simulink model "balancingController"  (Simulink 7.9)
settings: Solver=FixedStepDiscrete  StartTime=0.0  StopTime=60  FixedStep=Ts  RelTol=1e-3
InitFcn:
  | initBalancingController;
model workspace (MATLAB code in the model file):
  | Ts = 0.01;
undefined symbols (not defined in the file): DiscIntNeverNeededParam
libraries: WBCLibrary x12, simulink x2, dspsigops x2
settings Model: Creator=daniele  LastModifiedBy=morteza
settings DataIOCC: SignalLoggingSaveFormat=Dataset
settings SFSimCC: SimParseCustomCode=off
settings GRTTargetCC: CombineOutputUpdateFcns=off  GRTInterface=on

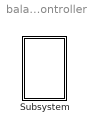
== system balancingController ==
  Subsystem : Subsystem  mask{robotName='icubGazeboSim', Ts=Ts, localName='dynamicBalancing'}
      mask prompts: robotName "robot name"; localName "module name"

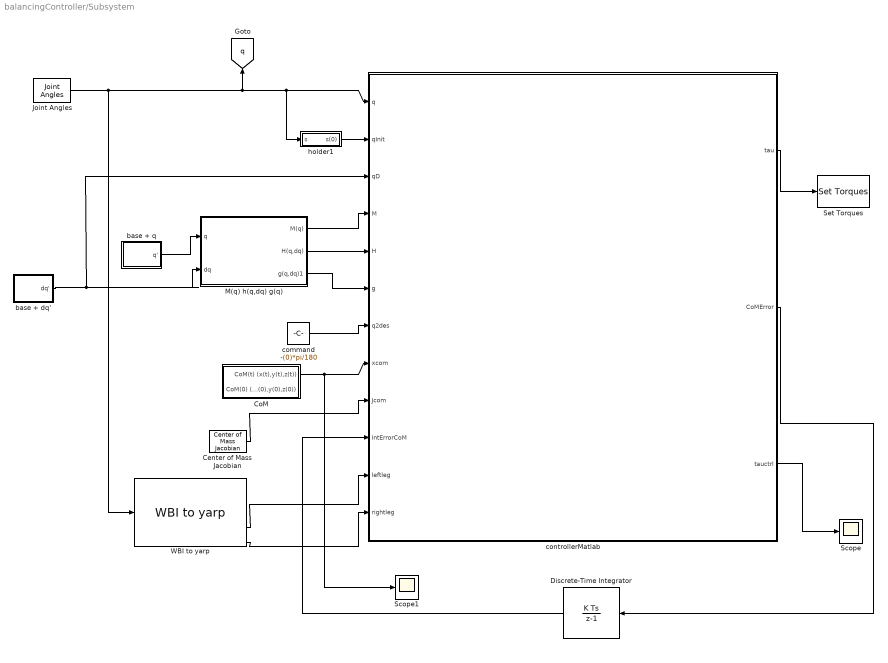
== system balancingController/Subsystem ==
  Center of Mass Jacobian : WBCLibrary/wholeBodyModel/Jacobians/Center of Mass Jacobian  robotName=robotName  localName=localName
  "CoM " : Subsystem
  Discrete-Time Integrator : DiscreteIntegrator  InitialCondition=[0 0 0]  SampleTime=Ts  ICPrevOutput=DiscIntNeverNeededParam  ICPrevScaledInput=DiscIntNeverNeededParam
  Joint Angles : WBCLibrary/wholeBodyStates/Joint Angles  robotName=robotName  localName=localName
  M(q) h(q,dq) g(q) : Subsystem
  Scope : Scope
      settings: YMin=16.125  YMax=16.325
  Scope1 : Scope
      settings: ShowLegends=on  YMin=-0.1  YMax=0.5
  Set Torques : WBCLibrary/wholeBodyActuators/Set Torques  val=6  robotName=robotName  localName=localName
  WBI to yarp : WBCLibrary/Utilities/WBI to yarp
  base + dq' : Subsystem
  base + q : Subsystem
  command : Constant  Value=-(0)*pi/180
  controllerMatlab : MATLAB Function  TreatAsAtomicUnit=on
  holder1 : Subsystem
  tag scope: q=global
  wires:
  Discrete-Time Integrator/1 -> controllerMatlab/10(IntErrorCoM)
  base + q/1(q') -> M(q) h(q,dq) g(q)/1(q)
  Joint Angles/1 -> [q], holder1/1(s), controllerMatlab/1(q), WBI to yarp/1
  controllerMatlab/2(CoMError) -> Discrete-Time Integrator/1
  M(q) h(q,dq) g(q)/1(M(q)) -> controllerMatlab/4(M)
  "CoM "/1(CoM(t) (x(t),y(t),z(t))) -> controllerMatlab/8(xcom), Scope1/1
  Center of Mass Jacobian/1 -> controllerMatlab/9(Jcom)
  holder1/1(s(0)) -> controllerMatlab/2(qInit)
  M(q) h(q,dq) g(q)/2(H(q,dq)) -> controllerMatlab/5(H)
  base + dq'/1(dq') -> M(q) h(q,dq) g(q)/2(dq), controllerMatlab/3(qD)
  command/1 -> controllerMatlab/7(q2des)
  WBI to yarp/4 -> controllerMatlab/11(leftleg)
  WBI to yarp/5 -> controllerMatlab/12(rightleg)
  controllerMatlab/1(tau) -> Set Torques/1
  M(q) h(q,dq) g(q)/3(g(q,dq)1) -> controllerMatlab/6(g)
  controllerMatlab/3(tauctrl) -> Scope/1

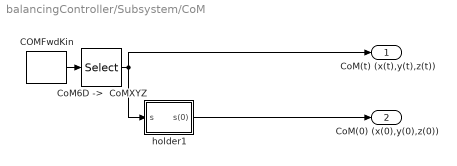
== system balancingController/Subsystem/CoM  ==
  "COMFwdKin " : WBCLibrary/wholeBodyModel/Forward Kinematics/COMFwdKin   robotName=robotName  localName=localName
  "CoM6D ->  CoMXYZ" : Selector  InputPortWidth=7  IndexOptions=Index vector (dialog)  Indices=[1 2 3]  OutputSizes=1
  holder1 : Subsystem
  CoM(t) (x(t),y(t),z(t)) : Outport
  CoM(0) (x(0),y(0),z(0)) : Outport  Port=2
  wires:
  "COMFwdKin "/1 -> "CoM6D ->  CoMXYZ"/1
  "CoM6D ->  CoMXYZ"/1 -> holder1/1(s), CoM(t) (x(t),y(t),z(t))/1
  holder1/1(s(0)) -> CoM(0) (x(0),y(0),z(0))/1

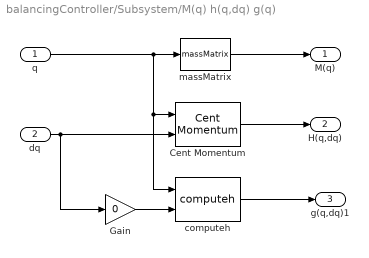
== system balancingController/Subsystem/M(q) h(q,dq) g(q) ==
  q : Inport
  dq : Inport  Port=2
  Cent Momentum : WBCLibrary/wholeBodyModel/Dynamics/Cent Momentum  robotName=robotName  localName=localName
  Gain : Gain  Gain=0
  computeh : WBCLibrary/wholeBodyModel/Dynamics/computeh  val=7  robotname=robotName  localname=localName
  massMatrix : WBCLibrary/wholeBodyModel/Dynamics/massMatrix  val=8  robotname=robotName  localname=localName
  M(q) : Outport
  H(q,dq) : Outport  Port=2
  g(q,dq)1 : Outport  Port=3
  wires:
  massMatrix/1 -> M(q)/1
  q/1 -> massMatrix/1, Cent Momentum/1, computeh/1
  Cent Momentum/1 -> H(q,dq)/1
  dq/1 -> Cent Momentum/2, Gain/1
  Gain/1 -> computeh/2
  computeh/1 -> g(q,dq)1/1

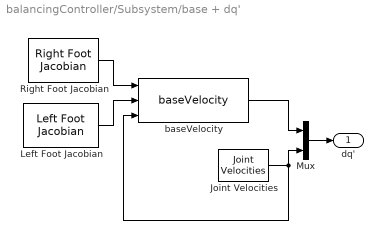
== system balancingController/Subsystem/base + dq' ==
  Joint Velocities : WBCLibrary/wholeBodyStates/Joint Velocities  robotName=robotName  localName=localName
  Left Foot Jacobian : WBCLibrary/wholeBodyModel/Jacobians/Left Foot Jacobian  robotName=robotName  localName=localName
  Mux : Mux  Inputs=2
  Right Foot Jacobian : WBCLibrary/wholeBodyModel/Jacobians/Right Foot Jacobian  robotName=robotName  localName=localName
  baseVelocity : WBCLibrary/Utilities/baseVelocity
  dq' : Outport
  wires:
  Left Foot Jacobian/1 -> baseVelocity/2
  Right Foot Jacobian/1 -> baseVelocity/1
  baseVelocity/1 -> Mux/1
  Joint Velocities/1 -> baseVelocity/3, Mux/2
  Mux/1 -> dq'/1

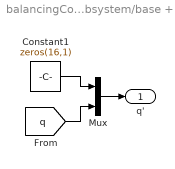
== system balancingController/Subsystem/base + q ==
  Constant1 : Constant  Value=zeros(16,1)
  Mux : Mux  Inputs=2
  q' : Outport
  wires:
  Mux/1 -> q'/1
  [q] -> Mux/2
  Constant1/1 -> Mux/1

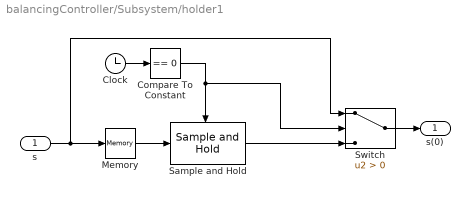
== system balancingController/Subsystem/holder1 ==
  s : Inport
  Clock : Clock
  Compare To Constant : simulink/Logic and Bit Operations/Compare To Constant  relop===  const=0  OutDataTypeStr=boolean
  Memory : Memory
  Sample and Hold : dspsigops/Sample and Hold  trig=Falling edge  initCond=0  latchinput=off
  Switch : Switch  Criteria=u2 > Threshold
  s(0) : Outport
  wires:
  s/1 -> Switch/1, Memory/1
  Clock/1 -> Compare To Constant/1
  Compare To Constant/1 -> Sample and Hold/Trigger, Switch/2
  Sample and Hold/1 -> Switch/3
  Switch/1 -> s(0)/1
  Memory/1 -> Sample and Hold/1

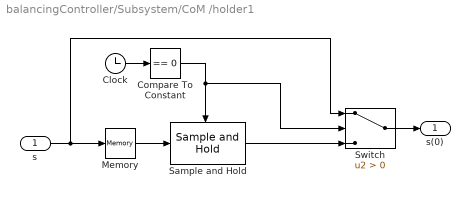
== system balancingController/Subsystem/CoM /holder1 ==
  s : Inport
  Clock : Clock
  Compare To Constant : simulink/Logic and Bit Operations/Compare To Constant  relop===  const=0  OutDataTypeStr=boolean
  Memory : Memory
  Sample and Hold : dspsigops/Sample and Hold  trig=Falling edge  initCond=0  latchinput=off
  Switch : Switch  Criteria=u2 > Threshold
  s(0) : Outport
  wires:
  s/1 -> Switch/1, Memory/1
  Clock/1 -> Compare To Constant/1
  Compare To Constant/1 -> Sample and Hold/Trigger, Switch/2
  Sample and Hold/1 -> Switch/3
  Switch/1 -> s(0)/1
  Memory/1 -> Sample and Hold/1

== matlab function Subsystem/controllerMatlab ==
  data: q input double; qInit input double; qD input double; M input double; H input double; g input double; q2des input double; tau output double; xcom input double; Jcom input double; CoMError output double; IntErrorCoM input double; leftleg input double; rightleg input double; tauctrl output double
function [tau,CoMError,tauctrl] = fcn(q,qInit,qD, M, H, g, q2des, xcom,Jcom, IntErrorCoM, leftleg, rightleg)
%#codegen


%% gain calculations
% gravity
grav_acc = 9.81;
% robot parameters
m1 = 11.948;
m2 = 10.2749;
l1 = 0.4366;
lc1 = 0.1911;
lc2 = 0.23;
I1 = 0.9356;
I2 = 0.1609;
% parameters of the motion Eqs.
c = m1 + m2;
c1 = m1*lc1^2 + m2*l1^2 + I1;
c2 = m2*lc2^2 + I2;
c3 = m2*l1*lc2;
c4 = m1*lc1 + m2*l1;
c5 = m2*lc2;
% desired final position
q2d = abs(q2des);
q1d = atan((c4+c5*cos(q2d))/(c5*sin(q2d)));
% The characteristic equation is
% a Z^4 + k1 Z^3 + (k2+beta+gamma1*ks) Z^2 + k3 Z + (gamma2*ks) = 0
% k1 = g K kdd,  k2 = g K kd,  k3 = g K kp
a = c1*c2 - c3^2*cos(q2d)^2;
K = c4*sin(q1d)*(c2+c3*cos(q2d)) - c5*sin(q1d+q2d)*(c1+c3*cos(q2d));
beta = grav_acc*(c3*c5*cos(q2d)*sin(q1d+q2d) - c2*c4*sin(q1d));
gamma1 = c1 + c2 + 2*c3*cos(q2d);
gamma2 = -grav_acc*(c4*sin(q1d) + c5*sin(q1d+q2d));
% (lambda + p)^4
p = 4;
ks = a*p^4/gamma2;
kp = 4*a*p^3/grav_acc/K;
kd = (6*a*p^2-beta-gamma1*ks)/grav_acc/K;
kdd = 4*a*p/grav_acc/K;

% kp = 23.1678;
% kd = 11.8792;
% kdd = 1.448;
% ks = -3.6625;
% c5 = 2.3635;

%% controller's calculations
% joint angles of the two-link robot
q1 = leftleg(5) + pi/2;     % =rightleg(5) + pi/2
q2 = -leftleg(1);       % =-rightleg(1);

% mass of the robot
m = M(1,1);
% velocity of the CoM
xDcom = Jcom(1:3,:)*qD;


xG = xcom(1);
xGd = xDcom(1);
ankle_height = 0.0685;
AngMom = H(4:6) + m*Sf(xcom)*xDcom - m*xDcom(1)*ankle_height;
L = -AngMom(2);
Ld = -m*grav_acc*xG;
Ldd = -m*grav_acc*xGd;
taug = c5*grav_acc*cos(q1+q2);
tauctrl = -(kp*L + kd*Ld + kdd*Ldd + ks*(q2des-q2) + taug);

% DoF
n = 25;
% St    = [zeros(6,n);eye(n,n)];

% Error of the CoM
CoMError    = xcom;
normCoMError  = norm(CoMError);

% zero torque for all joints
tau = zeros(n,1);

% active joint torque control
% tau(14) = tauctrl/2;
% tau(20) = tauctrl/2;
% passive joint torque control
% tau(18) = 0;
% tau(24) = 0;
